simulink model "Throttle_Map_Code_Generator"  (R2023b)
settings: Solver=FixedStepDiscrete  StartTime=0.0  StopTime=3180  FixedStep=0.015  RelTol=1e-3
settings Model: Creator=Inver  LastModifiedBy=Inver
settings DataIOCC: ExternalInput=ds_tm.getElement('rTVS'),ds_tm.getElement('rEQUAL'),ds_tm.getElement('V'),ds_tm.getElement('w'),ds_tm.getElement('TVS_STATE')  LoadExternalInput=on
settings OptimizationCC: DefaultParameterBehavior=Inlined  GainParamInheritBuiltInType=on  UseFloatMulNetSlope=on  UseSpecifiedMinMax=on  InlineInvariantSignals=on  StrengthReduction=on  PassReuseOutputArgsAs=Individual arguments  ZeroExternalMemoryAtStartup=off  ZeroInternalMemoryAtStartup=off  NoFixptDivByZeroProtection=on  EfficientFloat2IntCast=on  LifeSpan=1  OptimizeBlockOrder=speed  DifferentSizesBufferReuse=on  OptimizationPriority=Speed  MultiThreadedLoops=on  EfficientTunableParamExpr=on
settings DebuggingCC: ReadBeforeWriteMsg=DisableAll  WriteAfterWriteMsg=DisableAll  WriteAfterReadMsg=DisableAll  MultiTaskDSMMsg=none  ParameterTunabilityLossMsg=error
settings HardwareCC: ProdBitPerPointer=32  ProdBitPerSizeT=32  ProdBitPerPtrDiffT=32  ProdLargestAtomicInteger=Long  ProdLargestAtomicFloat=Double  ProdWordSize=32  ProdLongLongMode=on  ProdHWDeviceType=ARM Compatible->ARM Cortex-M
settings ModelReferenceCC: UpdateModelReferenceTargets=IfOutOfDate
settings SFSimCC: SFSimEcho=off  MATLABDynamicMemAlloc=off
settings RTWCC: Description=Embedded Coder  SystemTargetFile=ert.tlc  GenCodeOnly=on  PackageGeneratedCodeAndArtifacts=on  TemplateMakefile=ert_default_tmf  Toolchain=GNU Tools for ARM Embedded Processors  BuildConfiguration=Faster Runs
settings CodeAppCC: GenerateComments=off  IgnoreCustomStorageClasses=off  OperatorAnnotations=on  SimulinkDataObjDesc=on  SFDataObjDesc=on  SimulinkBlockComments=off
settings ERTTargetCC: TargetLangStandard=C99 (ISO)  GenerateSampleERTMain=on  CombineSignalStateStructs=on  SuppressErrorStatus=on  CodeInterfacePackaging=Reusable function  SupportNonFinite=off  SupportComplex=off  InlinedParameterPlacement=NonHierarchical  RootIOFormat=Structure reference  ERTCustomFileTemplate=example_file_process.tlc  GlobalDataDefinition=InSeparateSourceFile  DataDefinitionFile=data.c  GlobalDataReference=InSeparateHeaderFile  ERTFilePackagingFormat=CompactWithDataFile  DataReferenceFile=data.h

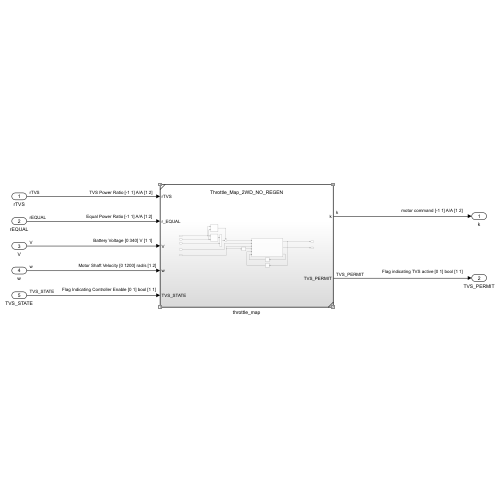
[thumbnail: Simulink's stored preview of the top-level diagram]
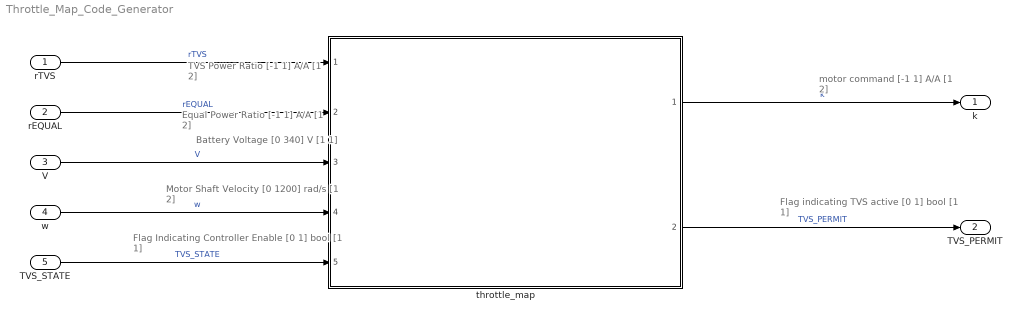
== system Throttle_Map_Code_Generator ==
  note: motor command [-1 1] A/A [1 2]
  note: Flag indicating TVS active [0 1] bool [1 1]
  note: Motor Shaft Velocity [0 1200] rad/s [1 2]
  note: Equal Power Ratio [-1 1] A/A [1 2]
  note: Battery Voltage [0 340] V [1 1]
  note: TVS Power Ratio [-1 1] A/A [1 2]
  note: Flag Indicating Controller Enable [0 1] bool [1 1]
  rTVS : Inport  PortDimensions=[1 2]
  rEQUAL : Inport  Port=2  PortDimensions=[1 2]
  V : Inport  Port=3  PortDimensions=[1 1]
  w : Inport  Port=4  PortDimensions=[1 2]
  TVS_STATE : Inport  Port=5  PortDimensions=[1 1]
  throttle_map : Subsystem  ReferencedSubsystem=Throttle_Map_2WD_NO_REGEN
  k : Outport
  TVS_PERMIT : Outport  Port=2
  wires:
  throttle_map/2 -> TVS_PERMIT/1  "TVS_PERMIT"
  throttle_map/1 -> k/1  "k"
  rEQUAL/1 -> throttle_map/2  "rEQUAL"
  rTVS/1 -> throttle_map/1  "rTVS"
  V/1 -> throttle_map/3  "V"
  w/1 -> throttle_map/4  "w"
  TVS_STATE/1 -> throttle_map/5  "TVS_STATE"
